simulink model "cosim"  (R2013b)
settings: Solver=FixedStepDiscrete  SolverMode=SingleTasking  StartTime=0.0  StopTime=inf  FixedStep=0.01  RelTol=1e-3
undefined symbols (not defined in the file): A, N
libraries: xbsIndex_r4 x11, simulink x4, JTAGRuntimeCosim_r4 x1
settings Model: Creator=laca  LastModifiedBy=laca

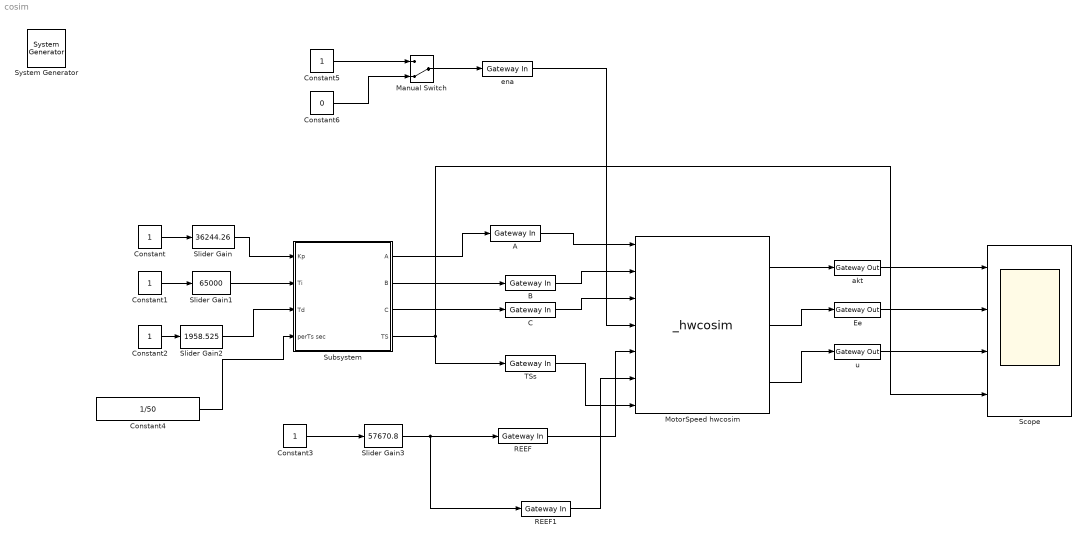
== system cosim ==
  " System Generator" : xbsIndex_r4/ System Generator  Tag=genX  xilinxfamily=spartan3e  part=xc3s500e  speed=-4  package=pq208  synthesis_tool=XST  clock_wrapper=Clock Enables  directory=./netlist  proj_type=Project Navigator  Synth_file=XST Defaults  Impl_file=ISE Defaults  testbench=off  simulink_period=1  sysclk_period=20  dcm_input_clock_period=10  incr_netlist=off  trim_vbits=Everywhere in SubSystem  dbl_ovrd=According to Block Masks  core_generation=According to Block Masks  run_coregen=off  deprecated_control=off  eval_field=0  block_type=sysgen
  A : xbsIndex_r4/Gateway In  gui_display_data_type=Fixed-point  arith_type=Unsigned  n_bits=16  bin_pt=0  preci_type=Single  exp_width=8  frac_width=24  quantization="Round  (unbiased: +/- Inf)"  overflow=Saturate  period=1  dbl_ovrd=off  timing_constraint=None  locs_specified=off  LOCs={}  UseAsADC=off  ADCChannel='1'  inherit_from_input=off  hdl_port=on  block_type=gatewayin
  B : xbsIndex_r4/Gateway In  gui_display_data_type=Fixed-point  arith_type=Unsigned  n_bits=16  bin_pt=0  preci_type=Single  exp_width=8  frac_width=24  quantization="Round  (unbiased: +/- Inf)"  overflow=Saturate  period=1  dbl_ovrd=off  timing_constraint=None  locs_specified=off  LOCs={}  UseAsADC=off  ADCChannel='1'  inherit_from_input=off  hdl_port=on  block_type=gatewayin
  C : xbsIndex_r4/Gateway In  gui_display_data_type=Fixed-point  arith_type=Unsigned  n_bits=16  bin_pt=0  preci_type=Single  exp_width=8  frac_width=24  quantization="Round  (unbiased: +/- Inf)"  overflow=Saturate  period=1  dbl_ovrd=off  timing_constraint=None  locs_specified=off  LOCs={}  UseAsADC=off  ADCChannel='1'  inherit_from_input=off  hdl_port=on  block_type=gatewayin
  Constant{,1..3,5} (5 alike) : Constant
  Constant4 : Constant  Value=1/50
  Constant6 : Constant  Value=0
  Ee : xbsIndex_r4/Gateway Out  inherit_from_input=off  hdl_port=on  timing_constraint=None  locs_specified=off  LOCs={}  UseAsDAC=off  DACChannel='1'  block_type=gatewayout
  Manual Switch : ManualSwitch  CurrentSetting=0
  MotorSpeed hwcosim : JTAGRuntimeCosim_r4/_hwcosim  clkSrc=Free Running  hasCombinationalPath=on  bitfileName=C:\Users\laca\Desktop\iRoobo2014Ver3\Fpga\SPARTAN3E\Spartan3E6500SystemVer2\dcMOTORVelocityPID\netlist\motorspeed_cw.bit  skipConfig=off  cable=Auto Detect  speed=N/A  cablePort=N/A  cableLocation=Local  shareCable=off  enable_codebug=on  design_xtable=|  engineDll=JTAGCosimEngine.dll  cableWaitTime=10  bscanPos=1  IRLengths=[6,8]  useWaitBox=1  hasBufgmux=on  Scheme=Cosim  useCmdProc=1  hasProc=0  useImpact=0  printLogFile=0  block_type=jtagcosim
      | {
      |   'clkWrapper' => 'motorspeed_cw',
      |   'clocksGcd' => undef,
      |   'device' => 'xc3s500e-4pq208',
      |   'ports' => {
      |     'aa' => {
      |       'bd_port_index' => 0,
      |       'direction' => 'in',
      |       'icon_text' => 'Aa',
      |       'period' => 1,
      |       'sim_pause_trigger' => false,
      |       'type' => 'UFix_16_0',
      |       'width' => 16,
      |     },
      |     'bb' => {
      |       'bd_port_index' => 1,
      |       'direction' => 'in',
      |       'icon_text' => 'Bb',
      |       'period' => 1,
      |       'sim_pause_trigger' => false,
      |       'type' => 'UFix_16_0',
      |       'width' => 16,
      |     },
      |     'cc' => {
      |       'bd_port_index' => 2,
      |       'direction' => 'in',
      |       'icon_text' => 'Cc',
      |       'period' => 1,
      |       'sim_pause_trigger' => false,
      |       'type' => 'UFix_16_0',
      |       'width' => 16,
      |     },
      |     'counterval' => {
      |       'bd_port_index' => 0,
      |       'direction' => 'out',
      |       'icon_text' => 'counterval',
      |       'period' => 1,
      |       'sim_pause_trigger' => false,
      |       'type' => 'Fix_16_0',
      |       'width' => 16,
      |     },
      |     'e' => {
      |       'bd_port_index' => 1,
      |       'direction' => 'out',
      |       'icon_text' => 'e',
      |       'period' => 1,
      |       'sim_pause_trigger' => false,
      |       'type' => 'Fix_17_0',
      |       'width' => 17,
      |     },
      |     'enapwm' => {
      |       'bd_port_index' => 3,
      |       'direction' => 'in',
      |       'icon_text' => 'enaPWM',
      |       'period' => 1,
      |       'sim_pause_trigger' => false,
      |       'type' => 'Bool',
      |       'width' => 1,
      |     },
      |     'gateway_in' => {
      |       'bd_port_index' => 4,
      |       'direction' => 'in',
      |       'icon_text' => 'Gateway In',
      |       'period' => 1,
      |       'sim_pause_trigger' => false,
      |       'type' => 'Fix_17_0',
      |       'width' => 17,
      |     },
      |     'recerencia' => {
      |       'bd_port_index' => 5,
      |       'direction' => 'in',
      |       'icon_text' => 'recerencia',
      |       'period' => 1,
      |       'sim_pause_trigger' => false,
      |       'type' => 'Fix_16_0',
      |       'width' => 16,
      |     },
      |     'ts' => {
      |       'bd_port_index' => 6,
      |       'direction' => 'in',
      |       'icon_text' => 'TS',
      |       'period' => 1,
      |       'sim_pause_trigger' => false,
      |       'type' => 'UFix_32_0',
      |       'width' => 32,
      |     },
      |     'u' => {
      |       'bd_port_index' => 2,
      |       'direction' => 'out',
      |       'icon_text' => 'u',
      |       'period' => 1,
      |       'sim_pause_trigger' => false,
      |       'type' => 'Fix_17_0',
      |       'width' => 17,
      |     },
      |   },
      |   'shared_memories' => {},
      | }
  REEF : xbsIndex_r4/Gateway In  gui_display_data_type=Fixed-point  arith_type="Signed  (2's comp)"  n_bits=17  bin_pt=0  preci_type=Single  exp_width=8  frac_width=24  quantization="Round  (unbiased: +/- Inf)"  overflow=Saturate  period=1  dbl_ovrd=off  timing_constraint=None  locs_specified=off  LOCs={}  UseAsADC=off  ADCChannel='1'  inherit_from_input=off  hdl_port=on  block_type=gatewayin
  REEF1 : xbsIndex_r4/Gateway In  gui_display_data_type=Fixed-point  arith_type="Signed  (2's comp)"  n_bits=16  bin_pt=0  preci_type=Single  exp_width=8  frac_width=24  quantization="Round  (unbiased: +/- Inf)"  overflow=Saturate  period=1  dbl_ovrd=off  timing_constraint=None  locs_specified=off  LOCs={}  UseAsADC=off  ADCChannel='1'  inherit_from_input=off  hdl_port=on  block_type=gatewayin
  Scope : Scope  NumInputPorts=4
      settings: YMin=3~-118~52500~678572  YMax=18~-103~67500~750000  SaveName=ScopeData2
  Slider Gain : simulink/Math Operations/Slider Gain  low=0  gain=36244.26  high=65000
  Slider Gain1 : simulink/Math Operations/Slider Gain  low=0  gain=65000  high=65000
  Slider Gain2 : simulink/Math Operations/Slider Gain  low=0  gain=1958.525  high=5000
  Slider Gain3 : simulink/Math Operations/Slider Gain  low=-65535  gain=57670.8  high=65535
  Subsystem : Subsystem
  TSs : xbsIndex_r4/Gateway In  gui_display_data_type=Fixed-point  arith_type=Unsigned  n_bits=32  bin_pt=0  preci_type=Single  exp_width=8  frac_width=24  quantization="Round  (unbiased: +/- Inf)"  overflow=Saturate  period=1  dbl_ovrd=off  timing_constraint=None  locs_specified=off  LOCs={}  UseAsADC=off  ADCChannel='1'  inherit_from_input=off  hdl_port=on  block_type=gatewayin
  akt : xbsIndex_r4/Gateway Out  inherit_from_input=off  hdl_port=on  timing_constraint=None  locs_specified=off  LOCs={}  UseAsDAC=off  DACChannel='1'  block_type=gatewayout
  ena : xbsIndex_r4/Gateway In  gui_display_data_type=Boolean  arith_type=Boolean  n_bits=16  bin_pt=0  preci_type=Single  exp_width=8  frac_width=24  quantization="Round  (unbiased: +/- Inf)"  overflow=Saturate  period=1  dbl_ovrd=off  timing_constraint=None  locs_specified=off  LOCs={}  UseAsADC=off  ADCChannel='1'  inherit_from_input=off  hdl_port=on  block_type=gatewayin
  u : xbsIndex_r4/Gateway Out  inherit_from_input=off  hdl_port=on  timing_constraint=None  locs_specified=off  LOCs={}  UseAsDAC=off  DACChannel='1'  block_type=gatewayout
  wires:
  MotorSpeed hwcosim/3 -> u/1
  Ee/1 -> Scope/2
  u/1 -> Scope/3
  Constant/1 -> Slider Gain/1
  Constant1/1 -> Slider Gain1/1
  Constant2/1 -> Slider Gain2/1
  A/1 -> MotorSpeed hwcosim/1
  C/1 -> MotorSpeed hwcosim/3
  B/1 -> MotorSpeed hwcosim/2
  Constant3/1 -> Slider Gain3/1
  REEF/1 -> MotorSpeed hwcosim/5
  MotorSpeed hwcosim/1 -> akt/1
  Subsystem/1(A) -> A/1
  Subsystem/2(B) -> B/1
  Subsystem/3(C) -> C/1
  Subsystem/4(TS) -> TSs/1, Scope/4
  Slider Gain/1 -> Subsystem/1(Kp)
  Slider Gain1/1 -> Subsystem/2(Ti)
  Slider Gain2/1 -> Subsystem/3(Td)
  Constant4/1 -> Subsystem/4(perTs sec)
  MotorSpeed hwcosim/2 -> Ee/1
  akt/1 -> Scope/1
  Slider Gain3/1 -> REEF1/1, REEF/1
  Constant5/1 -> Manual Switch/1
  Manual Switch/1 -> ena/1
  Constant6/1 -> Manual Switch/2
  ena/1 -> MotorSpeed hwcosim/4
  TSs/1 -> MotorSpeed hwcosim/7
  REEF1/1 -> MotorSpeed hwcosim/6

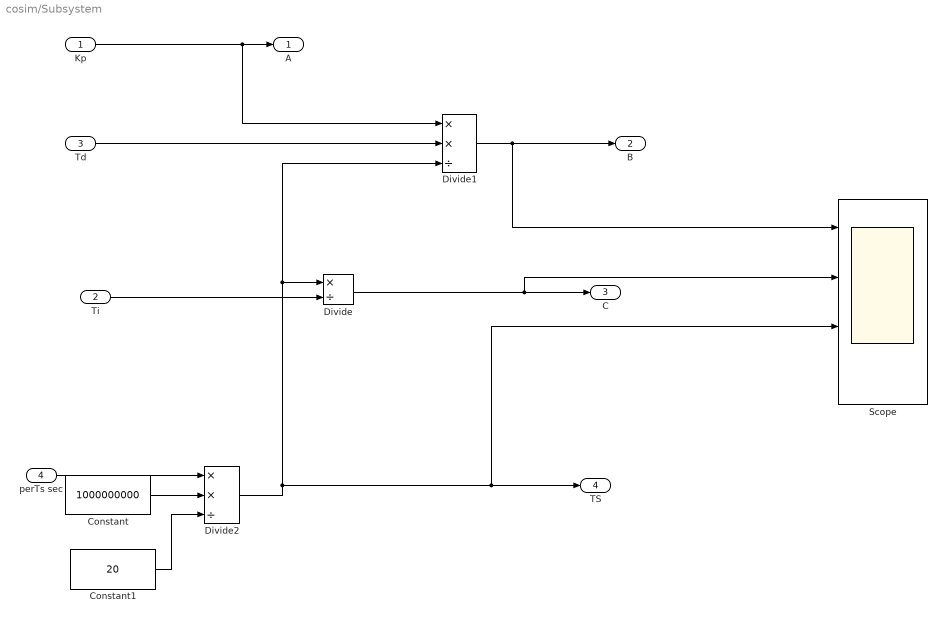
== system cosim/Subsystem ==
  Kp : Inport
  Ti : Inport  Port=2
  Td : Inport  Port=3
  perTs sec : Inport  Port=4
  Constant : Constant  Value=1000000000
  Constant1 : Constant  Value=20
  Divide : Product  Inputs=*/
  Divide1 : Product  Inputs=**/
  Divide2 : Product  Inputs=**/
  Scope : Scope  NumInputPorts=4
      settings: YMin=-1~-1~2375~-1  YMax=1~1~2625~1
  A : Outport
  B : Outport  Port=2
  C : Outport  Port=3
  TS : Outport  Port=4
  wires:
  Kp/1 -> Divide1/1, A/1
  Divide2/1 -> Scope/3, TS/1, Divide1/3, Divide/1
  perTs sec/1 -> Divide2/1
  Constant/1 -> Divide2/2
  Constant1/1 -> Divide2/3
  Divide/1 -> Scope/2, C/1
  Ti/1 -> Divide/2
  Td/1 -> Divide1/2
  Divide1/1 -> Scope/1, B/1
